simulink model "ctcsimulinkJan24"  (R2015a)
settings: Solver=ode45  StartTime=0.0  StopTime=6  RelTol=1e-3
libraries: dspindex x2, dspsrcs4 x1, dspvision x1, dspsnks4 x1
settings Model: Creator=User  LastModifiedBy=Madeline

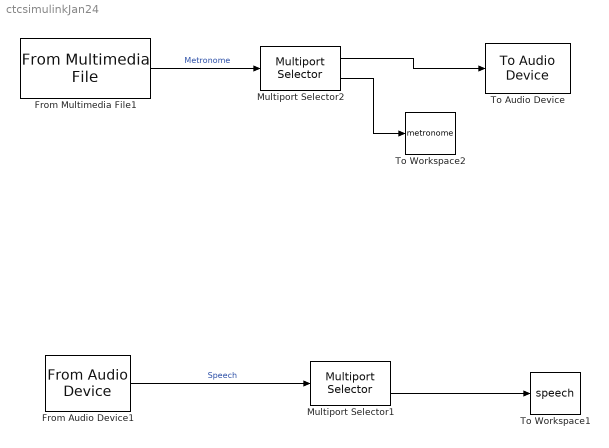
== system ctcsimulinkJan24 ==
  From Audio Device1 : dspsrcs4/From Audio Device  deviceName=Default  numChannels=2  sampleRate=44100  deviceDatatype=Determine from output data type  autoBufferSize=on  bufferSize=4096  queueDuration=1  frameSize=1024  outputDatatype=double  defaultInputChannelMapping=on  inputChannelMapping=1:2  outputNumOverrunSamples=off
  From Multimedia File1 : dspvision/From Multimedia File  inputFilename=C:\Users\Madeline\Documents\senior year (2015-2016)\spring 2016\senior design\senior design_matlab\tamborine_90bpm_4-4time_20beats_stereo_LEkFjP.mp3  loop=on  numPlays=1  outputStreams=Audio only  videoDataType=single  audioDataType=double  inheritSampleTime=on  userDefinedSampleTime=1/30  noAudioOutput=off  isIntensityVideo=off  fourcc=RGB  colorVideoFormat=Separate color signals  outputEOF=off  dataOrg=Column-major  audioFrameSize=1024  computeAudioFrameSize=off  outSamplingMode=Sample based
  Multiport Selector1 : dspindex/Multiport Selector  rowsOrCols=Columns  idxCellArray={1,2}  idxErrMode=Clip Index
  Multiport Selector2 : dspindex/Multiport Selector  rowsOrCols=Columns  idxCellArray={1,2}  idxErrMode=Clip Index
  To Audio Device : dspsnks4/To Audio Device  deviceName=Communications Headphones (IDT High Definition Audio CODEC)  inheritSampleRate=off  sampleRate=44100  deviceDatatype=Determine from input data type  autoBufferSize=on  bufferSize=4096  queueDuration=1.0  defaultOutputChannelMapping=on  outputChannelMapping=1:2  outputNumUnderrunSamples=off
  To Workspace1 : ToWorkspace  VariableName=speech  SampleTime=-1
      settings: Save2DSignal=2-D array (concatenate along first dimension)
  To Workspace2 : ToWorkspace  VariableName=metronome  SampleTime=-1
      settings: Save2DSignal=2-D array (concatenate along first dimension)
  wires:
  From Audio Device1/1 -> Multiport Selector1/1  "Speech"
  Multiport Selector1/2 -> To Workspace1/1
  From Multimedia File1/1 -> Multiport Selector2/1  "Metronome"
  Multiport Selector2/1 -> To Audio Device/1
  Multiport Selector2/2 -> To Workspace2/1
